simulink model "server"  (R2020a)
settings: Solver=FixedStepAuto  StartTime=0.0  StopTime=500  RelTol=1e-3
values from neighbouring files (symbols this model uses):
  n = 10    [Lab_1_kod.m]    (also in lab1.m)
undefined symbols (not defined in the file or in its folder): m
libraries: dspstat3 x1
settings Model: Creator=Bennu  LastModifiedBy=Piotr
settings DataIOCC: SaveOutput=off  SaveTime=off  ReturnWorkspaceOutputs=off
settings DebuggingCC: ArithmeticOperatorsInVariantConditions=warning
settings SFSimCC: SimUseLocalCustomCode=off  CustomCodeUndefinedFunction=UseInterfaceOnly
settings RTWCC: RTWUseLocalCustomCode=off
settings CodeAppCC: StateflowObjectComments=on

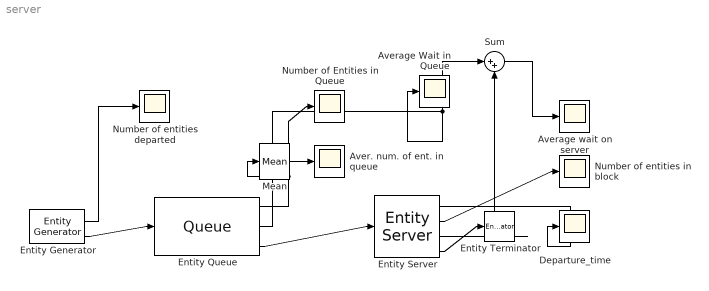
== system server ==
  Aver. num. of ent. in queue : Scope
  Average Wait in Queue : Scope
  Average wait on server : Scope
  Departure_time : Scope
  Entity Generator : EntityGenerator  OutputPortMessageModes=n,m  TimeSource=MATLAB action  IntergenerationTimeAction=|  GenerateEntityAtSimulationStart=off  GenerateAction=|  AttributeName=Number|PriorityA|Durations  AttributeInitialValue=0|0|0  NumberEntitiesDeparted=on  EntityType=Structured  EntityTypeName=Entity
      | % Pattern: Repeating Sequence
      | persistent A;
      | persistent idx;
      | if isempty(A)
      |     A = [4 38 28 30 23 22 45 36 84 12];
      |     idx = 1;
      | end
      | if idx > numel(A)
      |     dt = inf;
      | else
      |     dt = A(idx);
      | end
      | idx = idx + 1;
      | % Pattern: Repeating Sequence
      | persistent A;
      | persistent S;
      | persistent PRIO;
      | persistent idx;
      | if isempty(A)
      |     A = [1 2 3 4 5 6 7 8 9 10];
      |     S = [53 46 44 40 40 50 41 39 46 40];
      |     PRIO = [4 6 7 9 9 5 8 9 6 10];
      |     idx = 1;
      | end
      | if idx > numel(A)
      |     entity.Number = inf;
      |     entity.PriorityA = inf;
      |     entity.Durations = inf;
      | else
      |     entity.Number = A(idx);
      |     entity.PriorityA = PRIO(idx);
      |     entity.Durations = S(idx);
      | end
      | coder.extrinsic('assignin');
      | idx = idx + 1;
      settings: OutputPortMap=o0,o3
  Entity Queue : Queue  InputPortMessageModes=m  OutputPortMessageModes=n,n,m  Capacity=inf  QueueType=Priority  PrioritySource=PriorityA  SortingDirection=Descending  NumberEntitiesInBlock=on  AverageWait=on
      settings: OutputPortMap=o1,o2,o5
  Entity Server : EntityServer  InputPortMessageModes=m  OutputPortMessageModes=n,n,n,m  Capacity=1  ServiceTimeSource=Attribute  ServiceTimeAttributeName=Durations  ServiceTimeAction=|  NumberEntitiesDeparted=on  NumberEntitiesInBlock=on  AverageWait=on
      | % Pattern: Repeating Sequence
      | persistent SEQ;
      | persistent idx;
      | if isempty(SEQ)
      |     SEQ = [43 31 34 30 38 40 31 29 36 30];
      |     idx = 1;
      | end
      | if idx > numel(SEQ)
      |     dt = inf;
      | else
      |     dt = SEQ(idx);
      | end
      | idx = idx + 1;
      settings: OutputPortMap=o0,o1,o4,o9
  Entity Terminator : EntityTerminator  InputPortMessageModes=m  EntryAction=|
      | persistent idx;
      | persistent A;
      | coder.extrinsic('assignin');
      | if isempty(A)
      |     A = [0 0 0 0 0 0 0 0 0 0];
      |     idx = 1;
      | end
      | A(idx)=entity.Number;
      | if idx == 10
      |     assignin('base', 'order', A);
      | end
      | 
      | idx = idx+1;
  Mean : dspstat3/Mean  run=on  InputProcessing=Columns as channels (frame based)  reset_popup=None  directionMode=Entire input  dimension=1  roiEnable=off  roiType=Rectangles  roiPortion=Entire ROI  roiOutput=Individual statistics for each ROI  roiFlag=off  roundingMode=Floor  overflowMode=off  outputDataTypeStr=Inherit: Same as accumulator  outputMin=[]  outputMax=[]  outputLastDataTypeStr=Inherit: Same as accumulator
  Number of Entities in Queue : Scope
  Number of entities departed : Scope
  Number of entities in block : Scope
  Sum : Sum  Inputs=|++
  wires:
  Mean/1 -> Aver. num. of ent. in queue/1
  Entity Generator/1 -> Number of entities departed/1
  Sum/1 -> Average wait on server/1
  Entity Queue/3 -> Entity Server/1
  Entity Queue/1 -> Number of Entities in Queue/1, Mean/1
  Entity Server/3 -> Sum/2
  Entity Server/2 -> Number of entities in block/1
  Entity Queue/2 -> Sum/1, Average Wait in Queue/1
  Entity Server/4 -> Entity Terminator/1
  Entity Server/1 -> Departure_time/1
  Entity Generator/2 -> Entity Queue/1
